simulink library "equationsOfMotionSubsystem"  (R2021b)
settings: Solver=VariableStepAuto  StartTime=0.0  StopTime=10.0  RelTol=1e-3
undefined symbols (not defined in the file or in its folder): initialStateVector
libraries: equationsOfMotionLib x4, sharedutil x1
settings Model: Creator=mat  LastModifiedBy=mat

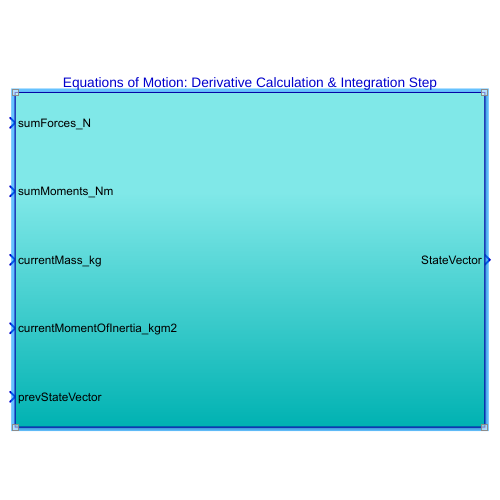
[thumbnail: Simulink's stored preview of the top-level diagram]
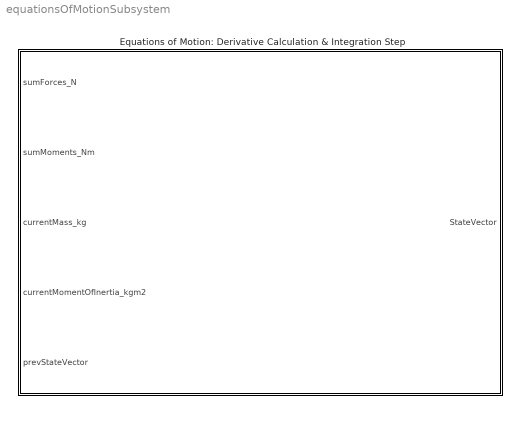
== system equationsOfMotionSubsystem ==
  Equations of Motion: Derivative Calculation & Integration Step : Subsystem

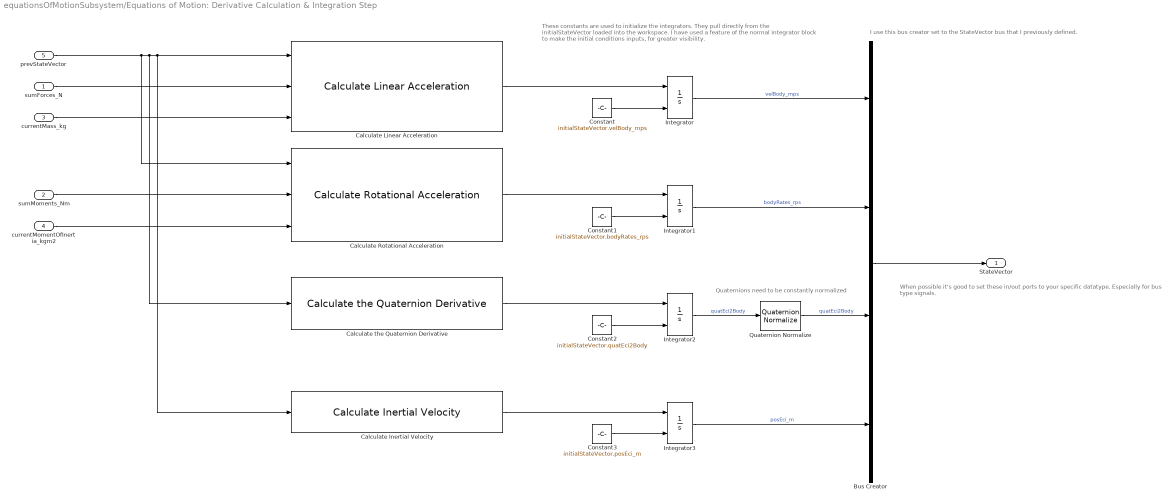
== system equationsOfMotionSubsystem/Equations of Motion: Derivative Calculation & Integration Step ==
  note: Quaternions need to be constantly normalized
  note: When possible it's good to set these in/out ports to your specific datatype. Especially for bus type signals.
  note: I use this bus creator set to the StateVector bus that I previously defined.
  note: These constants are used to initialize the integrators. They pull directly from the initialStateVector loaded into the workspace. I have used a feature of the normal integrator block to make the initial conditions inputs, for greater visibility.
  sumForces_N : Inport
  sumMoments_Nm : Inport  Port=2
  currentMass_kg : Inport  Port=3
  currentMomentOfInertia_kgm2 : Inport  Port=4
  prevStateVector : Inport  Port=5  OutDataTypeStr=Bus: StateVector_BusType
  Bus Creator : BusCreator  Inputs=4  OutDataTypeStr=Bus: StateVector_BusType  NonVirtualBus=on
      settings: InheritFromInputs=off
  Calculate Inertial Velocity : equationsOfMotionLib/Calculate Inertial Velocity  SystemSampleTime=-1  VariantActivationTime=update diagram  Latency=0  AutoFrameSizeCalculation=off
  Calculate Linear Acceleration : equationsOfMotionLib/Calculate Linear Acceleration  SystemSampleTime=-1  VariantActivationTime=update diagram  Latency=0  AutoFrameSizeCalculation=off
  Calculate Rotational Acceleration : equationsOfMotionLib/Calculate Rotational Acceleration  SystemSampleTime=-1  VariantActivationTime=update diagram  Latency=0  AutoFrameSizeCalculation=off
  Calculate the Quaternion Derivative : equationsOfMotionLib/Calculate the Quaternion Derivative  SystemSampleTime=-1  VariantActivationTime=update diagram  Latency=0  AutoFrameSizeCalculation=off
  Constant : Constant  Value=initialStateVector.velBody_mps
      settings: AttributesFormatString=%<Value>
  Constant1 : Constant  Value=initialStateVector.bodyRates_rps
      settings: AttributesFormatString=%<Value>
  Constant2 : Constant  Value=initialStateVector.quatEci2Body
      settings: AttributesFormatString=%<Value>
  Constant3 : Constant  Value=initialStateVector.posEci_m
      settings: AttributesFormatString=%<Value>
  Integrator{,1..3} (4 alike) : Integrator  InitialConditionSource=external
  Quaternion Normalize : sharedutil/Quaternion Normalize  aMode=aMode
      settings: SourceProductBaseCode=AE,PW,DR,MT,UV,VE
  StateVector : Outport  OutDataTypeStr=Bus: StateVector_BusType
  wires:
  prevStateVector/1 -> Calculate Rotational Acceleration/1, Calculate Linear Acceleration/1, Calculate Inertial Velocity/1, Calculate the Quaternion Derivative/1
  sumForces_N/1 -> Calculate Linear Acceleration/2
  currentMass_kg/1 -> Calculate Linear Acceleration/3
  Calculate Linear Acceleration/1 -> Integrator/1
  Constant/1 -> Integrator/2
  sumMoments_Nm/1 -> Calculate Rotational Acceleration/2
  currentMomentOfInertia_kgm2/1 -> Calculate Rotational Acceleration/3
  Calculate Rotational Acceleration/1 -> Integrator1/1
  Constant1/1 -> Integrator1/2
  Calculate the Quaternion Derivative/1 -> Integrator2/1
  Calculate Inertial Velocity/1 -> Integrator3/1
  Constant2/1 -> Integrator2/2
  Constant3/1 -> Integrator3/2
  Integrator/1 -> Bus Creator/1  "velBody_mps"
  Integrator1/1 -> Bus Creator/2  "bodyRates_rps"
  Integrator2/1 -> Quaternion Normalize/1  "quatEci2Body"
  Integrator3/1 -> Bus Creator/4  "posEci_m"
  Bus Creator/1 -> StateVector/1
  Quaternion Normalize/1 -> Bus Creator/3  "quatEci2Body"
